simulink model "simu3_pid"  (R2020b)
settings: Solver=VariableStepAuto  StartTime=0.0  StopTime=Ttt  MaxStep=0.2  RelTol=1e-3
values from neighbouring files (symbols this model uses):
  kd = 0.63    [lab3_4.m]
  ki = t_ki(j)    [lab3_2.m]    (also in lab3_4.m = 0.63; lab3_pi.m; test2.m = 0)
  kp = t_kp(i)    [lab3.m]    (also in lab3_2.m; lab3_4.m = 2.22; lab3_pi.m; test2.m = 1)
settings Model: Creator=pkubo  LastModifiedBy=pkubo
settings DataIOCC: ReturnWorkspaceOutputs=off

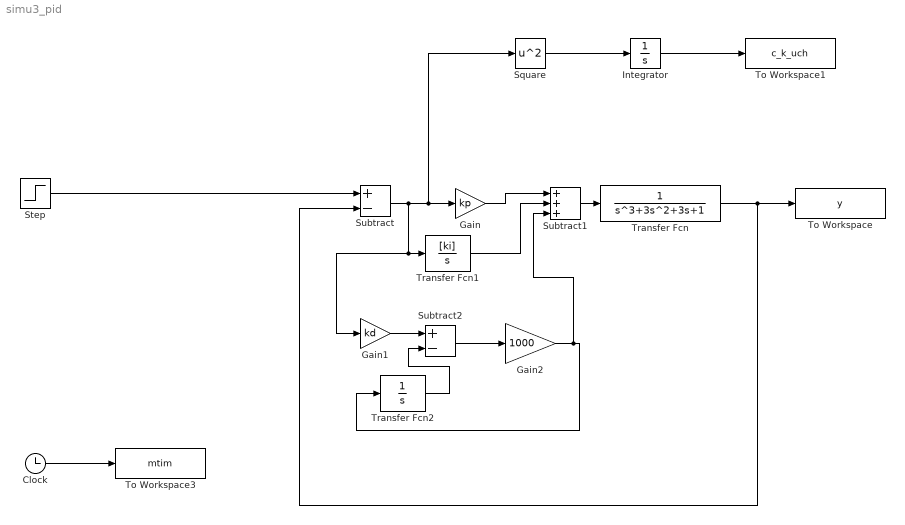
== system simu3_pid ==
  Clock : Clock
  Gain : Gain  Gain=kp
  Gain1 : Gain  Gain=kd
  Gain2 : Gain  Gain=1000
  Integrator : Integrator
  Square : Math  Operator=square  SignedPower=on  RndMeth=Zero  SaturateOnIntegerOverflow=on
  Step : Step  SampleTime=0
  Subtract : Sum  Inputs=+-
  Subtract1 : Sum  Inputs=+++
  Subtract2 : Sum  Inputs=+-
  To Workspace : ToWorkspace  VariableName=y  SampleTime=-1
  To Workspace1 : ToWorkspace  VariableName=c_k_uch  SampleTime=-1
  To Workspace3 : ToWorkspace  VariableName=mtim  SampleTime=-1
  Transfer Fcn : TransferFcn  Denominator=[1 3 3 1]
  Transfer Fcn1 : TransferFcn  Numerator=[ki]  Denominator=[1 0]
  Transfer Fcn2 : TransferFcn  Denominator=[1 0]
  wires:
  Transfer Fcn/1 -> Subtract/2, To Workspace/1
  Clock/1 -> To Workspace3/1
  Step/1 -> Subtract/1
  Integrator/1 -> To Workspace1/1
  Square/1 -> Integrator/1
  Subtract/1 -> Gain1/1, Transfer Fcn1/1, Gain/1, Square/1
  Gain/1 -> Subtract1/1
  Subtract1/1 -> Transfer Fcn/1
  Transfer Fcn1/1 -> Subtract1/2
  Gain1/1 -> Subtract2/1
  Transfer Fcn2/1 -> Subtract2/2
  Subtract2/1 -> Gain2/1
  Gain2/1 -> Subtract1/3, Transfer Fcn2/1
